simulink model "untitled"  (R2023a)
settings: Solver=VariableStepAuto  StartTime=0.0  StopTime=0.5  MaxStep=1e-3  RelTol=1e-3
libraries: cstblocks x2
settings Model: Creator=gnomy  LastModifiedBy=gnomy

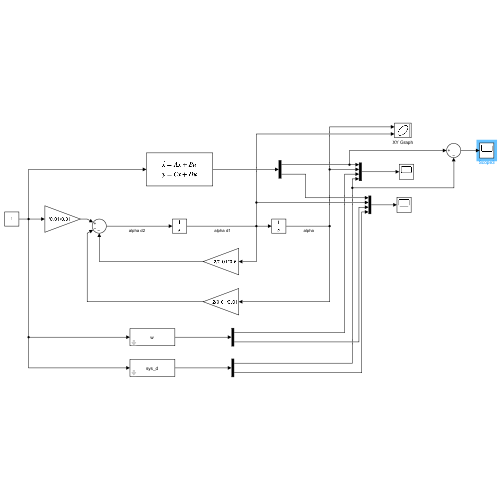
[thumbnail: Simulink's stored preview of the top-level diagram]
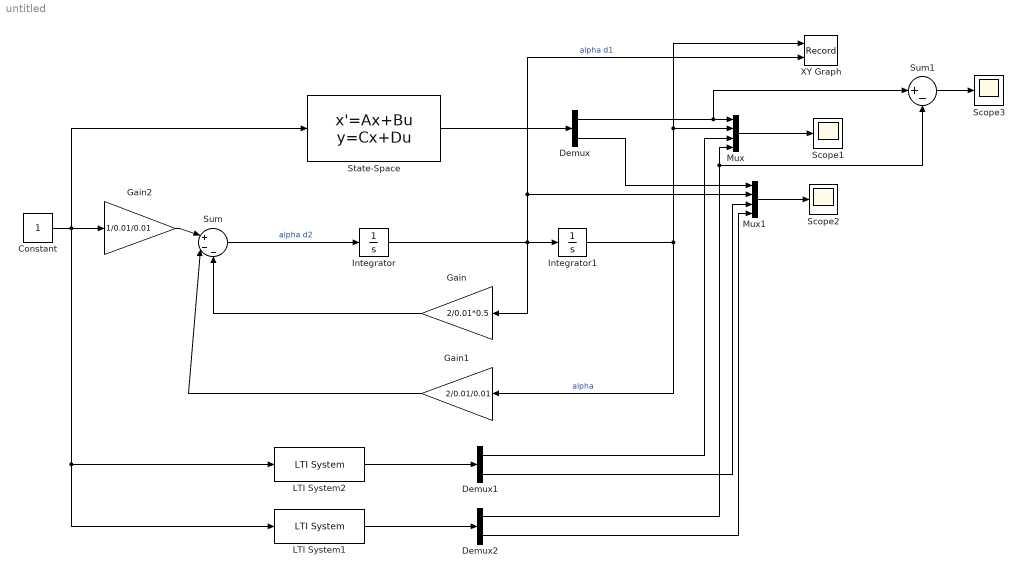
== system untitled ==
  Constant : Constant
  Demux : Demux  Outputs=2
  Demux1 : Demux  Outputs=2
  Demux2 : Demux  Outputs=2
  Gain : Gain  Gain=2/0.01*0.5
  Gain1 : Gain  Gain=2/0.01/0.01
  Gain2 : Gain  Gain=1/0.01/0.01
  Integrator : Integrator
  Integrator1 : Integrator
  LTI System1 : cstblocks/LTI System  sys=sys_d  IC=[]
  LTI System2 : cstblocks/LTI System  sys=w  IC=[]
  Mux : Mux
  Mux1 : Mux
  Scope1 : Scope
  Scope2 : Scope
  Scope3 : Scope
  State-Space : StateSpace  A=[0 1; -1/0.01^2 -2*0.5/0.01]  B=[0; 1/0.01^2]  C=[1 0; 0 1]  D=[0; 0]  InitialCondition=0
  Sum : Sum  Inputs=|+--
  Sum1 : Sum  Inputs=|+-
  XY Graph : Record  FileSettingsInternal="{\"entries\":[{\"content\":{\"excelSettings\":{\"content\":{},\"type\":\"Streamout.ExcelSettings\"}},\"type\":\"Streamout.FileSettingStorage\",\"uuid\":\"59f49d11-5cc8-4dad-b7d4-2d0f83484c7e\"}],\"packageUris\":[\"http://schema.mathworks.com/mf0/streamout_blocks/R2020a\"],\"version\":\"1.0\"}"  Layout=[1 1]  SignalsInternal="{\"entries\":[{\"content\":{\"signals\":[{\"content\":{\"blockPath\":[\"untitled/XY Graph\"],\"dimensions\":[1],\"domain\":\"untitled/XY Graph\",\"lineColor\":\"#a2142f\",\"plots\":[1],\"port\":1,\"sid\":[\"\"],\"signalID\":144,\"signalName\":\"alpha\"},\"type\":\"RecordBlkView.Signal\",\"uuid\":\"8206804b-b4a2-4681-9a01-21a6905e303a\"},{\"content\":{\"blockPath\":[\"untitled/XY Graph\"],\"dimensions\":[1],\"domain\":\"untitled/XY Graph\",\"lineColor\":\"#139fff\",\"plots\":[1],\"port\":2,\"sid\":[\"\"],\"signalID\":148,\"signalName\":\"alpha d1\"},\"type\":\"RecordBlkView.Signal\",\"uuid\":\"847cd8f6-32fa-4dc0-90e0-f3aed54eccee\"}]},\"type\":\"RecordBlkView.InputSignals\",\"uuid\":\"d648f33d-5bf9-4b08-8d6b-19544c57e7b4\"}],\"packageUris\":[\"http://schema.mathworks.com/mf0/streamout_blocks/R2020a\"],\"version\":\"1.0\"}"  VisualizationBindings="{\"xyplotplugin\":{\"info\":[{\"series\":[{\"bindingParametersList\":[{\"parameter\":\"X-Axis\",\"signalID\":144,\"signalName\":\"alpha\"},{\"parameter\":\"Y-Axis\",\"signalID\":148,\"signalName\":\"alpha d1\"}],\"seriesID\":29527}],\"subplotID\":1}]}}"  CompatibilityTag=XY
  wires:
  Sum/1 -> Integrator/1  "alpha d2"
  Integrator/1 -> Gain/1, XY Graph/2, Mux1/2, Integrator1/1  "alpha d1"
  Integrator1/1 -> Gain1/1, XY Graph/1, Mux/2  "alpha"
  Gain/1 -> Sum/3
  Gain1/1 -> Sum/2
  State-Space/1 -> Demux/1
  Demux/1 -> Sum1/1, Mux/1
  Mux/1 -> Scope1/1
  Constant/1 -> LTI System1/1, LTI System2/1, State-Space/1, Gain2/1
  Gain2/1 -> Sum/1
  Demux/2 -> Mux1/1
  Mux1/1 -> Scope2/1
  LTI System2/1 -> Demux1/1
  LTI System1/1 -> Demux2/1
  Demux1/1 -> Mux/3
  Demux2/1 -> Sum1/2, Mux/4
  Demux1/2 -> Mux1/3
  Demux2/2 -> Mux1/4
  Sum1/1 -> Scope3/1
